simulink model "rfpsc_parallel"  (R2023b)
settings: Solver=VariableStepAuto  StartTime=0  StopTime=1.5  FixedStep=0.1*T_s  RelTol=1e-4  AbsTol=1e-4  EnableMultiTasking=on
StopFcn:
  | save('../converter-testing/sim.mat', 'u_c2', 'i_c2', 'u_c2_ref_lim', 'p_c2', 'q_c2', 'i_c2_ref', 'p_c2_ref', 'q_c2_ref', 'u_c1', 'i_c1', 'u_c1_ref_lim', 'p_c1', 'q_c1', 'i_c1_ref', 'p_c1_ref', 'q_c1_ref', 'u_pcc', 'i_g', 'u_hat_pcc', 'p_hat_g', 'q_hat_g', 'u_pcc_abc', 'i_g_abc', 'theta_g', 'theta_c2');
undefined symbols (not defined in the file): f_sw, K_p, kpp, L_f1, L_f2, L_g, R_a, R_f, R_f1, R_f2, R_L, T_s, U_dc, u_gN, w0_pll, w_b, w_g, w_N
libraries: simulink x2
settings Model: Creator=mhinkkan  LastModifiedBy=chowd
settings SolverCC: AutoScaleAbsTol=off  MaxConsecutiveMinStep=10  AlgebraicLoopSolver=TrustRegion
settings DataIOCC: SaveFormat=Array  SignalLoggingSaveFormat=ModelDataLogs  SaveOutput=off  SignalLogging=off  DSMLogging=off  ReturnWorkspaceOutputs=off
settings OptimizationCC: BlockReduction=off  BooleanDataType=off  DefaultParameterBehavior=Inlined  OptimizeBlockIOStorage=off  BufferReuse=off  ReuseModelBlockBuffer=off  ExpressionFolding=off  ExpressionDepthLimit=2147483647  LocalBlockOutputs=off  InitFltsAndDblsToZero=on  LifeSpan=inf
settings DebuggingCC: AlgebraicLoopMsg=none  SaveWithParameterizedLinksMsg=none  UnderspecifiedInitializationDetection=Classic  MergeDetectMultiDrivingBlocksExec=none  SignalResolutionControl=TryResolveAllWithWarning  MultiTaskDSMMsg=warning  MultiTaskCondExecSysMsg=none  FcnCallInpInsideContextMsg=warning  UnconnectedInputMsg=warning  UnconnectedOutputMsg=warning  UnconnectedLineMsg=warning  StateNameClashWarn=warning  SFUnexpectedBacktrackingDiag=warning  SFNoUnconditionalDefaultTransitionDiag=warning  SFExecutionAtInitializationDiag=none  ArithmeticOperatorsInVariantConditions=warning
settings HardwareCC: ProdBitPerPointer=32  ProdBitPerSizeT=32  ProdBitPerPtrDiffT=32  ProdLargestAtomicFloat=None  ProdIntDivRoundTo=Undefined  ProdEndianess=Unspecified  ProdWordSize=32  ProdHWDeviceType=32-bit Generic  TargetUnknown=on
settings ModelReferenceCC: PropagateSignalLabelsOutOfModel=off
settings SFSimCC: SimUseLocalCustomCode=off  CustomCodeUndefinedFunction=UseInterfaceOnly
settings RTWCC: RTWUseLocalCustomCode=off
settings CodeAppCC: StateflowObjectComments=on
settings GRTTargetCC: TargetFcnLib=ansi_tfl_tmw.mat  TargetLangStandard=C89/C90 (ANSI)  CombineOutputUpdateFcns=off  GRTInterface=on
settings ConfigComp: CovMetricSettings=dw  CovSaveCumulativeToWorkspaceVar=on  CovSaveSingleToWorkspaceVar=on  CovExternalEMLEnable=off

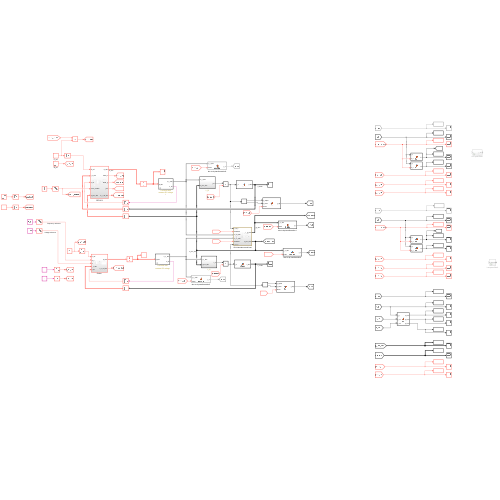
[thumbnail: Simulink's stored preview of the top-level diagram]
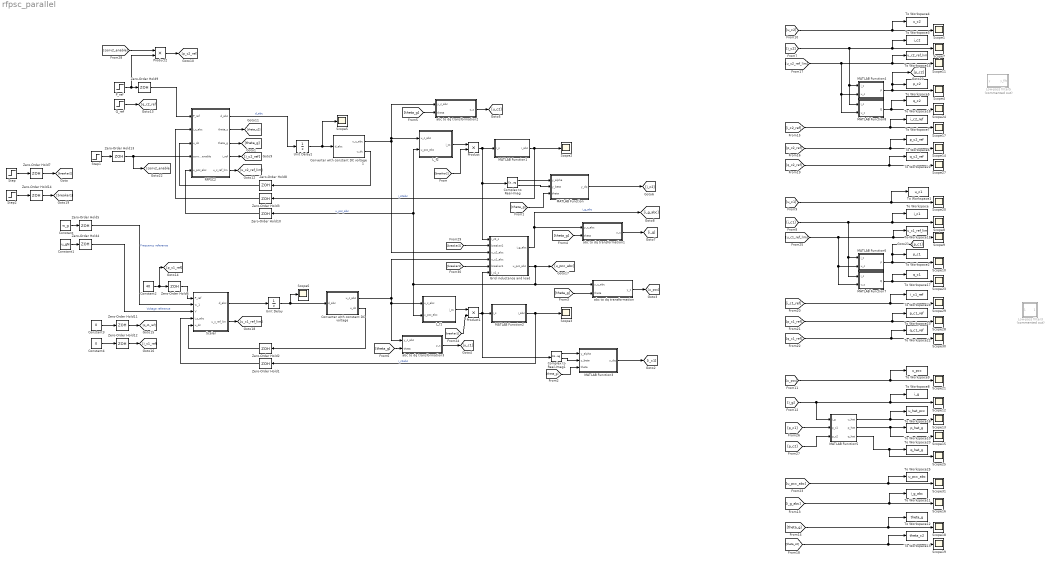
== system rfpsc_parallel ==
  Complex to Real-Imag : ComplexToRealImag
  Complex to Real-Imag1 : ComplexToRealImag
  Constant : Constant  Value=w_g
  Constant1 : Constant  Value=u_gN
  Constant2 : Constant  Value=40  SampleTime=T_s
  Constant3 : Constant  Value=0
  Constant4 : Constant  Value=0
  "Converter with constant DC voltage " : Subsystem  mask{f_sw=f_sw, u_dc=U_dc}
      mask prompts: f_sw "Switching frequency (Hz)"; u_dc "DC-bus voltage (V)"
      mask init:
      | T_s = 1/(2*f_sw);
  Converter with constant DC voltage 1 : Subsystem  mask{f_sw=f_sw, u_dc=U_dc}
      mask prompts: f_sw "Switching frequency (Hz)"; u_dc "DC-bus voltage (V)"
      mask init:
      | T_s = 1/(2*f_sw);
  Grid inductance and load : Subsystem
  L_f1 : Subsystem
  L_f2 : Subsystem
  Low-pass filter3 : Subsystem  Commented=on
  Low-pass filter5 : Subsystem  Commented=on
  MATLAB Function : MATLAB Function  TreatAsAtomicUnit=on
  MATLAB Function1 : MATLAB Function  TreatAsAtomicUnit=on
  MATLAB Function2 : MATLAB Function  TreatAsAtomicUnit=on
  MATLAB Function3 : MATLAB Function  TreatAsAtomicUnit=on
  MATLAB Function4 : MATLAB Function  TreatAsAtomicUnit=on
  MATLAB Function5 : MATLAB Function  TreatAsAtomicUnit=on
  MATLAB Function6 : MATLAB Function  TreatAsAtomicUnit=on
  MATLAB Function7 : MATLAB Function  TreatAsAtomicUnit=on
  MATLAB Function8 : MATLAB Function  TreatAsAtomicUnit=on
  P_ref : Step  Time=.9  Before=10  After=20  SampleTime=T_s
  Product : Product
  Product1 : Product
  Product2 : Product
  Q_ref : Step  Time=.35  After=0  SampleTime=T_s
  RFPSC2 : Subsystem
  "Scaler " : Subsystem
  Scope{1..21,23..25,27..31} (29 alike) : Scope
  Step : Step  Time=.3  SampleTime=T_s
  Step1 : Step  Time=.6  SampleTime=T_s
  Step2 : Step  Time=1.2  Before=1  After=0  SampleTime=T_s
  To Workspace : ToWorkspace  VariableName=i_c1  SaveFormat=Timeseries  SampleTime=-1
  To Workspace1 : ToWorkspace  VariableName=u_c1  SaveFormat=Timeseries  SampleTime=-1
  To Workspace10 : ToWorkspace  VariableName=p_hat_g  SaveFormat=Timeseries  SampleTime=-1
  To Workspace11 : ToWorkspace  VariableName=i_g_abc  SaveFormat=Timeseries  SampleTime=-1
  To Workspace12 : ToWorkspace  VariableName=theta_g  SaveFormat=Timeseries  SampleTime=-1
  To Workspace13 : ToWorkspace  VariableName=theta_c2  SaveFormat=Timeseries  SampleTime=-1
  To Workspace14 : ToWorkspace  VariableName=u_c2_ref_lim  SaveFormat=Timeseries  SampleTime=-1
  To Workspace15 : ToWorkspace  VariableName=u_c1_ref_lim  SaveFormat=Timeseries  SampleTime=-1
  To Workspace16 : ToWorkspace  VariableName=u_hat_pcc  SaveFormat=Timeseries  SampleTime=-1
  To Workspace17 : ToWorkspace  VariableName=q_c1  SaveFormat=Timeseries  SampleTime=-1
  To Workspace18 : ToWorkspace  VariableName=q_c2  SaveFormat=Timeseries  SampleTime=-1
  To Workspace2 : ToWorkspace  VariableName=p_c1  SaveFormat=Timeseries  SampleTime=-1
  To Workspace20 : ToWorkspace  VariableName=q_hat_g  SaveFormat=Timeseries  SampleTime=-1
  To Workspace21 : ToWorkspace  VariableName=q_c2_ref  SaveFormat=Timeseries  SampleTime=-1
  To Workspace22 : ToWorkspace  VariableName=q_c1_ref  SaveFormat=Timeseries  SampleTime=-1
  To Workspace23 : ToWorkspace  VariableName=p_c1_ref  SaveFormat=Timeseries  SampleTime=-1
  To Workspace24 : ToWorkspace  VariableName=i_c1_ref  SaveFormat=Timeseries  SampleTime=-1
  To Workspace25 : ToWorkspace  VariableName=u_pcc_abc  SaveFormat=Timeseries  SampleTime=-1
  To Workspace3 : ToWorkspace  VariableName=i_c2  SaveFormat=Timeseries  SampleTime=-1
  To Workspace4 : ToWorkspace  VariableName=u_c2  SaveFormat=Timeseries  SampleTime=-1
  To Workspace5 : ToWorkspace  VariableName=p_c2  SaveFormat=Timeseries  SampleTime=-1
  To Workspace6 : ToWorkspace  VariableName=p_c2_ref  SaveFormat=Timeseries  SampleTime=-1
  To Workspace7 : ToWorkspace  VariableName=i_c2_ref  SaveFormat=Timeseries  SampleTime=-1
  To Workspace8 : ToWorkspace  VariableName=i_g  SaveFormat=Timeseries  SampleTime=-1
  To Workspace9 : ToWorkspace  VariableName=u_pcc  SaveFormat=Timeseries  SampleTime=-1
  Unit Delay : UnitDelay  SampleTime=T_s  HasFrameUpgradeWarning=on
  Unit Delay1 : UnitDelay  SampleTime=T_s  HasFrameUpgradeWarning=on
  Zero-Order Hold{1..14} (14 alike) : ZeroOrderHold  SampleTime=T_s
  abc to dq transformation : MATLAB Function  TreatAsAtomicUnit=on
  abc to dq transformation1 : MATLAB Function  TreatAsAtomicUnit=on
  abc to dq transformation2 : MATLAB Function  TreatAsAtomicUnit=on
  abc to dq transformation3 : MATLAB Function  TreatAsAtomicUnit=on
  wires:
  Grid inductance and load/1(i_g_abc) -> [i_g_abc], abc to dq transformation1/1(y_c_abc)  "i_g_abc"
  Product1/1 -> Grid inductance and load/6(i_c1_s), Complex to Real-Imag1/1, MATLAB Function2/1(i_s)
  MATLAB Function2/1(i_abc) -> Scope3/1, Zero-Order Hold1/1  "i_c1abc"
  Grid inductance and load/2(u_pcc_abc) -> Zero-Order Hold10/1, L_f2/2(u_pcc_abc), L_f1/2(u_pcc_abc), abc to dq transformation/1(y_c_abc), [u_pcc_abc]  "u_pcc_abc"
  "Converter with constant DC voltage "/2(u_dc) -> Zero-Order Hold2/1
  "Scaler "/1(d_abc) -> Unit Delay/1
  Zero-Order Hold4/1 -> "Scaler "/3(V)  "Voltage reference"
  Constant1/1 -> Zero-Order Hold4/1
  Unit Delay/1 -> "Converter with constant DC voltage "/1(d_abc), Scope6/1
  Constant/1 -> Zero-Order Hold5/1
  Zero-Order Hold5/1 -> "Scaler "/2(w_1)  "Frequency reference"
  "Converter with constant DC voltage "/1(u_c_abc) -> abc to dq transformation3/1(y_c_abc), L_f1/1(u_c_abc), Grid inductance and load/4(u_c1_abc)
  Converter with constant DC voltage 1/1(u_c_abc) -> L_f2/1(u_c_abc), abc to dq transformation2/1(y_c_abc), Grid inductance and load/3(u_c2_abc)
  Unit Delay1/1 -> Scope5/1, Converter with constant DC voltage 1/1(d_abc)
  P_ref/1 -> Zero-Order Hold9/1, Product2/2
  Zero-Order Hold9/1 -> RFPSC2/1(P_ref)
  Converter with constant DC voltage 1/2(u_dc) -> Zero-Order Hold8/1
  MATLAB Function1/1(i_abc) -> Zero-Order Hold3/1, Scope2/1  "i_c2abc"
  Zero-Order Hold8/1 -> RFPSC2/3(u_dc)
  Zero-Order Hold3/1 -> RFPSC2/2(i_c_abc)
  Zero-Order Hold2/1 -> "Scaler "/5(u_dc)
  Zero-Order Hold1/1 -> "Scaler "/4(i_c_abc)
  Constant2/1 -> [p_c1_ref], Zero-Order Hold6/1
  Zero-Order Hold6/1 -> "Scaler "/1(P_ref)
  Step/1 -> Zero-Order Hold7/1
  Zero-Order Hold7/1 -> [breaker2]
  RFPSC2/1(d_abc) -> Unit Delay1/1  "d_abc"
  Product/1 -> Complex to Real-Imag/1, Grid inductance and load/1(i_c2_s), MATLAB Function1/1(i_s)
  L_f2/1(i_cs) -> Product/1
  [breaker2] -> Product/2
  Complex to Real-Imag/1 -> MATLAB Function/1(y_alpha)
  Complex to Real-Imag/2 -> MATLAB Function/2(y_beta)
  [theta_g] -> MATLAB Function/3(theta)
  Complex to Real-Imag1/1 -> MATLAB Function3/1(y_alpha)
  Complex to Real-Imag1/2 -> MATLAB Function3/2(y_beta)
  [theta_g] -> MATLAB Function3/3(theta)
  MATLAB Function3/1(y_dq) -> [i_c1]
  [theta_g] -> abc to dq transformation/2(theta)
  [theta_g] -> abc to dq transformation1/2(theta)
  [theta_g] -> abc to dq transformation2/2(theta)
  [theta_g] -> abc to dq transformation3/2(theta)
  Zero-Order Hold10/1 -> RFPSC2/5(u_pcc_abc)
  RFPSC2/3(theta_g) -> [theta_g]
  abc to dq transformation/1(y_c) -> [u_pcc]
  abc to dq transformation3/1(y_c) -> [u_c1]
  abc to dq transformation2/1(y_c) -> [u_c2]
  MATLAB Function/1(y_dq) -> [i_c2]
  abc to dq transformation1/1(y_c) -> [i_g]
  [i_c1] -> To Workspace/1, Scope8/1, MATLAB Function7/1(i_c), MATLAB Function6/1(i_c)
  RFPSC2/4(i_ref) -> [i_c2_ref]
  RFPSC2/2(theta_c) -> [theta_c2]
  RFPSC2/5(u_c_ref_lim) -> [u_c2_ref_lim]
  MATLAB Function6/1(P) -> To Workspace2/1, [p_c1], Scope10/1
  MATLAB Function4/1(P) -> [p_c2], To Workspace5/1, Scope4/1
  [i_c2] -> To Workspace3/1, Scope7/1, MATLAB Function8/1(i_c), MATLAB Function4/1(i_c)
  [p_c2_ref] -> To Workspace6/1, Scope14/1
  MATLAB Function5/2(p_hat) -> Scope15/1, To Workspace10/1
  [i_g_abc] -> To Workspace11/1, Scope16/1
  [i_c2_ref] -> To Workspace7/1, Scope17/1
  [theta_g] -> To Workspace12/1, Scope18/1
  [theta_c2] -> To Workspace13/1, Scope19/1
  MATLAB Function7/1(Q) -> To Workspace17/1, Scope23/1
  MATLAB Function8/1(Q) -> To Workspace18/1, Scope24/1
  MATLAB Function5/3(q_hat) -> Scope25/1, To Workspace20/1
  Q_ref/1 -> [q_c2_ref]
  [q_c2_ref] -> To Workspace21/1, Scope27/1
  [q_c1_ref] -> Scope30/1, To Workspace22/1
  [i_c1_ref] -> Scope29/1, To Workspace24/1
  [p_c1_ref] -> Scope28/1, To Workspace23/1
  Constant3/1 -> Zero-Order Hold11/1
  Constant4/1 -> Zero-Order Hold12/1
  [u_c1_ref_lim] -> To Workspace15/1, Scope9/1, MATLAB Function6/2(u_c), MATLAB Function7/2(u_c)
  [u_c2_ref_lim] -> To Workspace14/1, Scope11/1, MATLAB Function8/2(u_c), MATLAB Function4/2(u_c)
  [u_pcc_abc] -> To Workspace25/1, Scope31/1
  Zero-Order Hold11/1 -> [q_c1_ref]
  Zero-Order Hold12/1 -> [i_c1_ref]
  "Scaler "/2(u_c_ref_lim) -> [u_c1_ref_lim]
  Step1/1 -> Zero-Order Hold13/1
  Zero-Order Hold13/1 -> [conv2_enable], RFPSC2/4(conv_enable)
  Zero-Order Hold14/1 -> [breaker1]
  Step2/1 -> Zero-Order Hold14/1
  L_f1/1(i_cs) -> Product1/1
  [breaker1] -> Product1/2
  [u_c2] -> To Workspace4/1, Scope1/1
  [u_c1] -> To Workspace1/1, Scope20/1
  [u_pcc] -> Scope21/1, To Workspace9/1
  [i_g] -> MATLAB Function5/1(i_g), To Workspace8/1, Scope12/1
  MATLAB Function5/1(u_hat) -> To Workspace16/1, Scope13/1
  [p_c1] -> MATLAB Function5/2(p_c1)
  [p_c2] -> MATLAB Function5/3(p_c2)
  [conv2_enable] -> Product2/1
  Product2/1 -> [p_c2_ref]
  [breaker2] -> Grid inductance and load/2(breaker2)
  [breaker1] -> Grid inductance and load/5(breaker1)

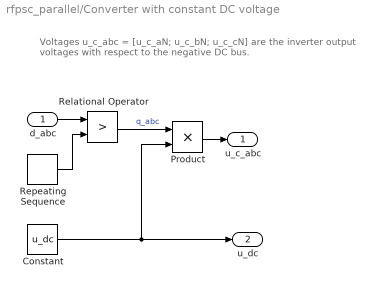
== system rfpsc_parallel/Converter with constant DC voltage  ==
  note: Voltages u_c_abc = [u_c_aN; u_c_bN; u_c_cN] are the inverter
      | output voltages with respect to the negative DC bus.
  d_abc : Inport
  Constant : Constant  Value=u_dc
  Product : Product
  Relational Operator : RelationalOperator  Operator=>  OutDataTypeStr='double'  InputSameDT=off
  Repeating Sequence : simulink/Sources/Repeating Sequence  rep_seq_t=[0 1 2]*T_s  rep_seq_y=[1 0 1]
  u_c_abc : Outport
  u_dc : Outport  Port=2
  wires:
  Repeating Sequence/1 -> Relational Operator/2
  d_abc/1 -> Relational Operator/1
  Product/1 -> u_c_abc/1
  Relational Operator/1 -> Product/1  "q_abc"
  Constant/1 -> Product/2, u_dc/1

== system rfpsc_parallel/Converter with constant DC voltage 1 ==
  note: Voltages u_c_abc = [u_c_aN; u_c_bN; u_c_cN] are the inverter
      | output voltages with respect to the negative DC bus.
  d_abc : Inport
  Constant : Constant  Value=u_dc
  Product : Product
  Relational Operator : RelationalOperator  Operator=>  OutDataTypeStr='double'  InputSameDT=off
  Repeating Sequence : simulink/Sources/Repeating Sequence  rep_seq_t=[0 1 2]*T_s  rep_seq_y=[1 0 1]
  u_c_abc : Outport
  u_dc : Outport  Port=2
  wires:
  Constant/1 -> u_dc/1, Product/2
  Relational Operator/1 -> Product/1  "q_abc"
  Product/1 -> u_c_abc/1
  d_abc/1 -> Relational Operator/1
  Repeating Sequence/1 -> Relational Operator/2

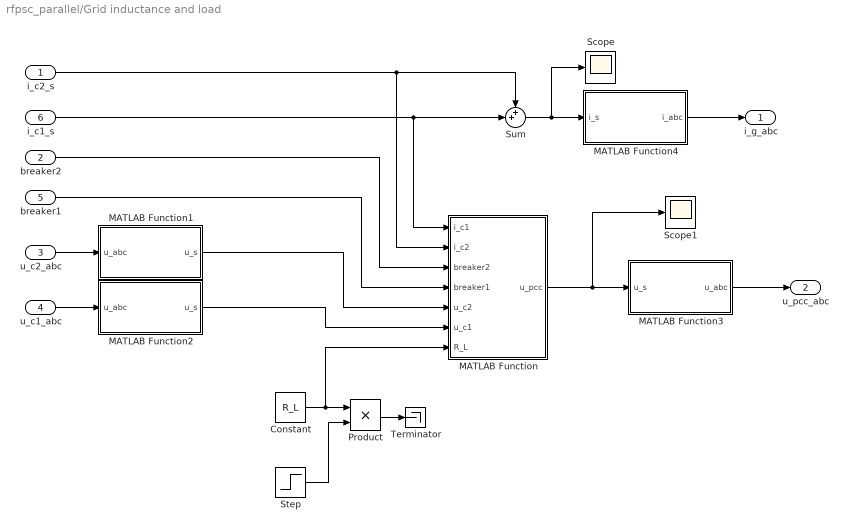
== system rfpsc_parallel/Grid inductance and load ==
  i_c2_s : Inport
  breaker2 : Inport  Port=2
  u_c2_abc : Inport  Port=3
  u_c1_abc : Inport  Port=4
  breaker1 : Inport  Port=5
  i_c1_s : Inport  Port=6
  Constant : Constant  Value=R_L  SampleTime=-1
  MATLAB Function : MATLAB Function  TreatAsAtomicUnit=on
  MATLAB Function1 : MATLAB Function  TreatAsAtomicUnit=on
  MATLAB Function2 : MATLAB Function  TreatAsAtomicUnit=on
  MATLAB Function3 : MATLAB Function  TreatAsAtomicUnit=on
  MATLAB Function4 : MATLAB Function  TreatAsAtomicUnit=on
  Product : Product
  Scope : Scope
  Scope1 : Scope
  Step : Step  Time=.06  Before=1  After=0.5  SampleTime=T_s
  Sum : Sum  Inputs=++|
  Terminator : Terminator
  i_g_abc : Outport
  u_pcc_abc : Outport  Port=2
  wires:
  Sum/1 -> MATLAB Function4/1(i_s), Scope/1
  i_c2_s/1 -> Sum/1, MATLAB Function/2(i_c2)
  i_c1_s/1 -> MATLAB Function/1(i_c1), Sum/2
  u_c2_abc/1 -> MATLAB Function1/1(u_abc)
  u_c1_abc/1 -> MATLAB Function2/1(u_abc)
  MATLAB Function1/1(u_s) -> MATLAB Function/5(u_c2)
  MATLAB Function2/1(u_s) -> MATLAB Function/6(u_c1)
  MATLAB Function/1(u_pcc) -> Scope1/1, MATLAB Function3/1(u_s)
  MATLAB Function3/1(u_abc) -> u_pcc_abc/1
  MATLAB Function4/1(i_abc) -> i_g_abc/1
  Step/1 -> Product/2
  Constant/1 -> MATLAB Function/7(R_L), Product/1
  Product/1 -> Terminator/1
  breaker2/1 -> MATLAB Function/3(breaker2)
  breaker1/1 -> MATLAB Function/4(breaker1)

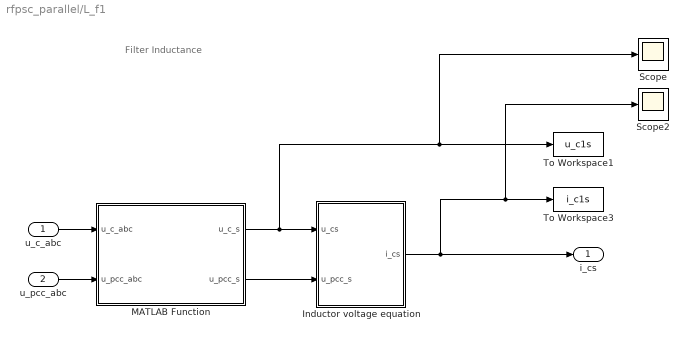
== system rfpsc_parallel/L_f1 ==
  note: Filter Inductance
  u_c_abc : Inport
  u_pcc_abc : Inport  Port=2
  Inductor voltage equation : Subsystem
  MATLAB Function : MATLAB Function  TreatAsAtomicUnit=on
  Scope : Scope
  Scope2 : Scope
  To Workspace1 : ToWorkspace  VariableName=u_c1s  SaveFormat=Timeseries
  To Workspace3 : ToWorkspace  VariableName=i_c1s  SaveFormat=Timeseries
  i_cs : Outport
  wires:
  Inductor voltage equation/1(i_cs) -> i_cs/1, Scope2/1, To Workspace3/1
  MATLAB Function/1(u_c_s) -> Inductor voltage equation/1(u_cs), Scope/1, To Workspace1/1
  u_c_abc/1 -> MATLAB Function/1(u_c_abc)
  MATLAB Function/2(u_pcc_s) -> Inductor voltage equation/2(u_pcc_s)
  u_pcc_abc/1 -> MATLAB Function/2(u_pcc_abc)

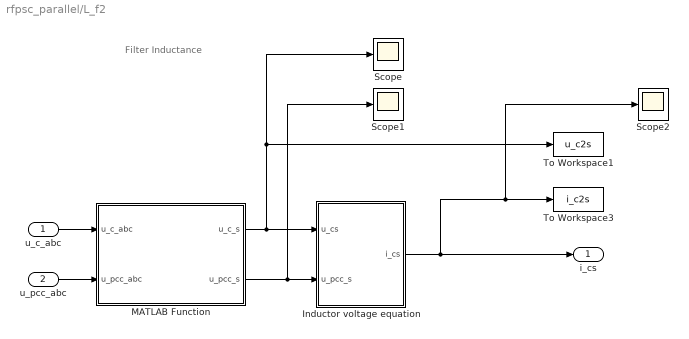
== system rfpsc_parallel/L_f2 ==
  note: Filter Inductance
  u_c_abc : Inport
  u_pcc_abc : Inport  Port=2
  Inductor voltage equation : Subsystem
  MATLAB Function : MATLAB Function  TreatAsAtomicUnit=on
  Scope : Scope
  Scope1 : Scope
  Scope2 : Scope
  To Workspace1 : ToWorkspace  VariableName=u_c2s  SaveFormat=Timeseries
  To Workspace3 : ToWorkspace  VariableName=i_c2s  SaveFormat=Timeseries
  i_cs : Outport
  wires:
  Inductor voltage equation/1(i_cs) -> i_cs/1, Scope2/1, To Workspace3/1
  MATLAB Function/1(u_c_s) -> Inductor voltage equation/1(u_cs), To Workspace1/1, Scope/1
  u_c_abc/1 -> MATLAB Function/1(u_c_abc)
  MATLAB Function/2(u_pcc_s) -> Scope1/1, Inductor voltage equation/2(u_pcc_s)
  u_pcc_abc/1 -> MATLAB Function/2(u_pcc_abc)

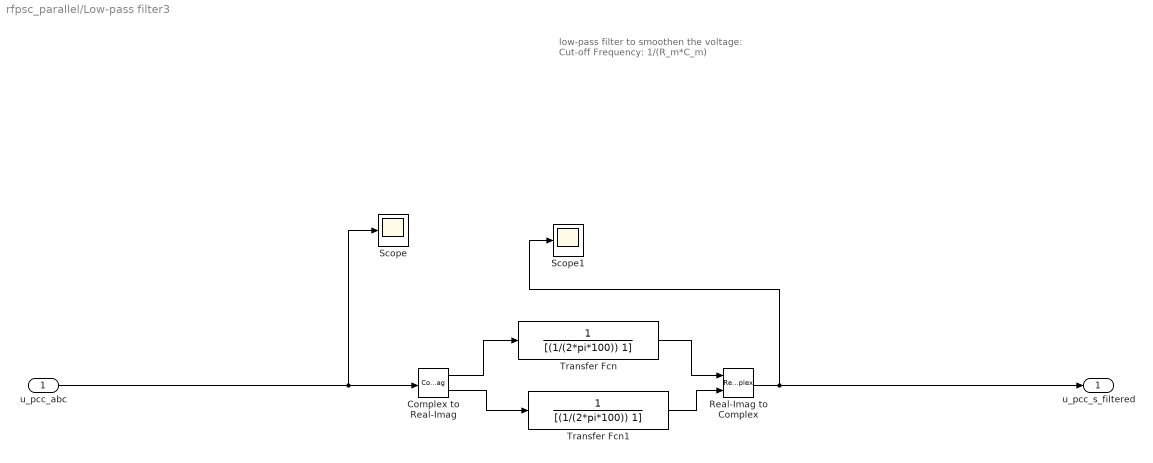
== system rfpsc_parallel/Low-pass filter3 ==
  note: low-pass filter to smoothen the voltage:
      | Cut-off Frequency: 1/(R_m*C_m)
  u_pcc_abc : Inport
  Complex to Real-Imag : ComplexToRealImag
  Real-Imag to Complex : RealImagToComplex
  Scope : Scope
  Scope1 : Scope
  Transfer Fcn : TransferFcn  Denominator=[(1/(2*pi*100)) 1]
  Transfer Fcn1 : TransferFcn  Denominator=[(1/(2*pi*100)) 1]
  u_pcc_s_filtered : Outport
  wires:
  Transfer Fcn1/1 -> Real-Imag to Complex/2
  Real-Imag to Complex/1 -> u_pcc_s_filtered/1, Scope1/1
  Complex to Real-Imag/1 -> Transfer Fcn/1
  u_pcc_abc/1 -> Complex to Real-Imag/1, Scope/1
  Transfer Fcn/1 -> Real-Imag to Complex/1
  Complex to Real-Imag/2 -> Transfer Fcn1/1

== system rfpsc_parallel/Low-pass filter5 ==
  note: low-pass filter to smoothen the voltage:
      | Cut-off Frequency: 1/(R_m*C_m)
  y : Inport
  Complex to Real-Imag : ComplexToRealImag
  Real-Imag to Complex : RealImagToComplex
  Transfer Fcn : TransferFcn  Denominator=[(1/(2*pi*1100)) 1]
  Transfer Fcn1 : TransferFcn  Denominator=[(1/(2*pi*1100)) 1]
  y_filt : Outport
  wires:
  Real-Imag to Complex/1 -> y_filt/1
  y/1 -> Complex to Real-Imag/1
  Transfer Fcn/1 -> Real-Imag to Complex/2
  Transfer Fcn1/1 -> Real-Imag to Complex/1
  Complex to Real-Imag/2 -> Transfer Fcn/1
  Complex to Real-Imag/1 -> Transfer Fcn1/1

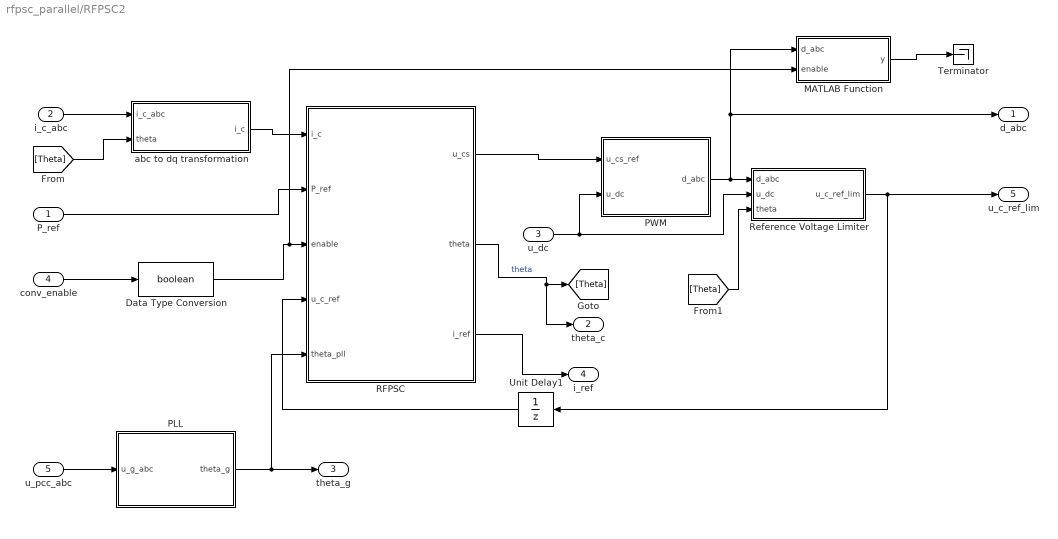
== system rfpsc_parallel/RFPSC2 ==
  P_ref : Inport
  i_c_abc : Inport  Port=2
  u_dc : Inport  Port=3
  conv_enable : Inport  Port=4
  u_pcc_abc : Inport  Port=5
  Data Type Conversion : DataTypeConversion  OutDataTypeStr=boolean  SaturateOnIntegerOverflow=off  RndMeth=Floor
  MATLAB Function : MATLAB Function  TreatAsAtomicUnit=on
  PLL : Subsystem
  PWM : Subsystem
  RFPSC : Subsystem
  Reference Voltage Limiter : Subsystem
  Terminator : Terminator
  Unit Delay1 : UnitDelay  SampleTime=T_s  HasFrameUpgradeWarning=on
  abc to dq transformation : MATLAB Function  TreatAsAtomicUnit=on  SystemSampleTime=T_s
  d_abc : Outport
  theta_c : Outport  Port=2
  theta_g : Outport  Port=3
  i_ref : Outport  Port=4
  u_c_ref_lim : Outport  Port=5
  wires:
  conv_enable/1 -> Data Type Conversion/1
  [Theta] -> Reference Voltage Limiter/3(theta)
  PWM/1(d_abc) -> d_abc/1, MATLAB Function/1(d_abc), Reference Voltage Limiter/1(d_abc)
  RFPSC/1(u_cs) -> PWM/1(u_cs_ref)
  Unit Delay1/1 -> RFPSC/4(u_c_ref)
  P_ref/1 -> RFPSC/2(P_ref)
  abc to dq transformation/1(i_c) -> RFPSC/1(i_c)
  Reference Voltage Limiter/1(u_c_ref_lim) -> Unit Delay1/1, u_c_ref_lim/1
  u_dc/1 -> Reference Voltage Limiter/2(u_dc), PWM/2(u_dc)
  [Theta] -> abc to dq transformation/2(theta)
  RFPSC/2(theta) -> theta_c/1, [Theta]  "theta"
  i_c_abc/1 -> abc to dq transformation/1(i_c_abc)
  PLL/1(theta_g) -> RFPSC/5(theta_pll), theta_g/1
  u_pcc_abc/1 -> PLL/1(u_g_abc)
  Data Type Conversion/1 -> MATLAB Function/2(enable), RFPSC/3(enable)
  MATLAB Function/1(y) -> Terminator/1
  RFPSC/3(i_ref) -> i_ref/1

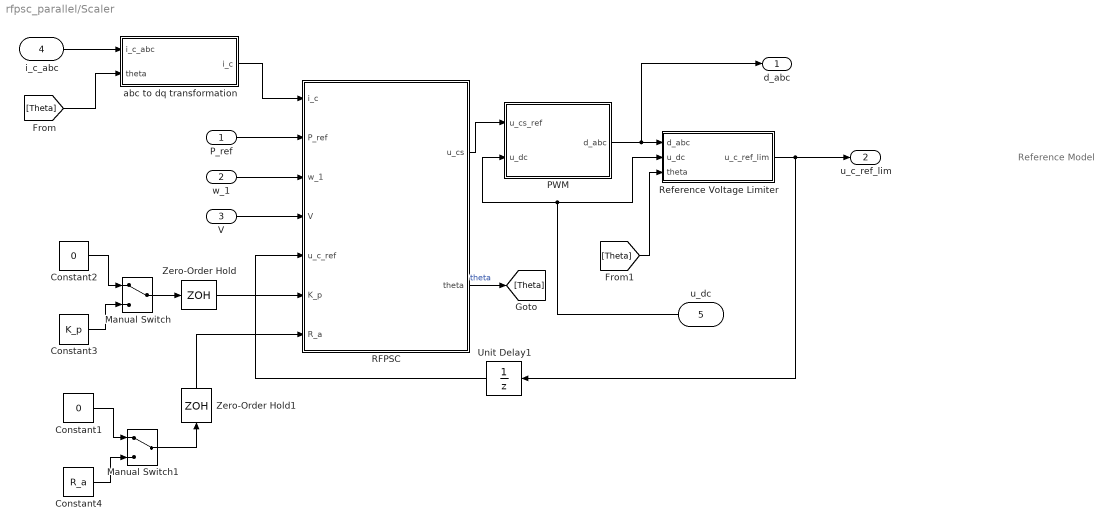
== system rfpsc_parallel/Scaler  ==
  note: Reference Model
  P_ref : Inport
  w_1 : Inport  Port=2
  V : Inport  Port=3
  i_c_abc : Inport  Port=4
  u_dc : Inport  Port=5
  Constant1 : Constant  Value=0  SampleTime=T_s
  Constant2 : Constant  Value=0  SampleTime=T_s
  Constant3 : Constant  Value=K_p  SampleTime=T_s
  Constant4 : Constant  Value=R_a  SampleTime=T_s
  Manual Switch : ManualSwitch
  Manual Switch1 : ManualSwitch
  PWM : Subsystem
  RFPSC : Subsystem
  Reference Voltage Limiter : Subsystem
  Unit Delay1 : UnitDelay  SampleTime=-1  HasFrameUpgradeWarning=on
  Zero-Order Hold : ZeroOrderHold  SampleTime=T_s
  Zero-Order Hold1 : ZeroOrderHold  SampleTime=T_s
  abc to dq transformation : MATLAB Function  TreatAsAtomicUnit=on
  d_abc : Outport
  u_c_ref_lim : Outport  Port=2
  wires:
  w_1/1 -> RFPSC/3(w_1)
  abc to dq transformation/1(i_c) -> RFPSC/1(i_c)
  Unit Delay1/1 -> RFPSC/5(u_c_ref)
  [Theta] -> abc to dq transformation/2(theta)
  [Theta] -> Reference Voltage Limiter/3(theta)
  Reference Voltage Limiter/1(u_c_ref_lim) -> Unit Delay1/1, u_c_ref_lim/1
  P_ref/1 -> RFPSC/2(P_ref)
  i_c_abc/1 -> abc to dq transformation/1(i_c_abc)
  PWM/1(d_abc) -> d_abc/1, Reference Voltage Limiter/1(d_abc)
  V/1 -> RFPSC/4(V)
  u_dc/1 -> PWM/2(u_dc), Reference Voltage Limiter/2(u_dc)
  RFPSC/1(u_cs) -> PWM/1(u_cs_ref)
  RFPSC/2(theta) -> [Theta]  "theta"
  Constant4/1 -> Manual Switch1/2
  Constant2/1 -> Manual Switch/1
  Manual Switch1/1 -> Zero-Order Hold1/1
  Constant1/1 -> Manual Switch1/1
  Constant3/1 -> Manual Switch/2
  Manual Switch/1 -> Zero-Order Hold/1
  Zero-Order Hold/1 -> RFPSC/6(K_p)
  Zero-Order Hold1/1 -> RFPSC/7(R_a)

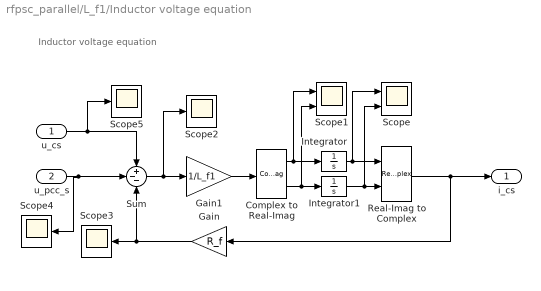
== system rfpsc_parallel/L_f1/Inductor voltage equation ==
  note: Inductor voltage equation
  u_cs : Inport
  u_pcc_s : Inport  Port=2
  Complex to Real-Imag : ComplexToRealImag
  Gain : Gain  Gain=R_f
  Gain1 : Gain  Gain=1/L_f1
  Integrator : Integrator
  Integrator1 : Integrator
  Real-Imag to Complex : RealImagToComplex
  Scope : Scope  NumInputPorts=2
  Scope1 : Scope  NumInputPorts=2
  Scope{2..5} (4 alike) : Scope
  Sum : Sum  Inputs=+--
  i_cs : Outport
  wires:
  Gain/1 -> Scope3/1, Sum/3
  Real-Imag to Complex/1 -> i_cs/1, Gain/1
  Integrator1/1 -> Real-Imag to Complex/2, Scope/2
  Integrator/1 -> Real-Imag to Complex/1, Scope/1
  Complex to Real-Imag/2 -> Integrator1/1, Scope1/2
  Complex to Real-Imag/1 -> Integrator/1, Scope1/1
  Gain1/1 -> Complex to Real-Imag/1
  Sum/1 -> Scope2/1, Gain1/1
  u_pcc_s/1 -> Scope4/1, Sum/2
  u_cs/1 -> Scope5/1, Sum/1

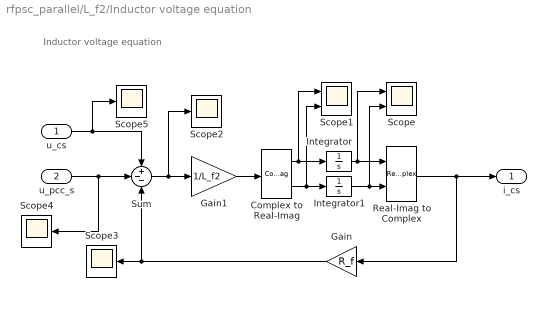
== system rfpsc_parallel/L_f2/Inductor voltage equation ==
  note: Inductor voltage equation
  u_cs : Inport
  u_pcc_s : Inport  Port=2
  Complex to Real-Imag : ComplexToRealImag
  Gain : Gain  Gain=R_f
  Gain1 : Gain  Gain=1/L_f2
  Integrator : Integrator
  Integrator1 : Integrator
  Real-Imag to Complex : RealImagToComplex
  Scope : Scope  NumInputPorts=2
  Scope1 : Scope  NumInputPorts=2
  Scope{2..5} (4 alike) : Scope
  Sum : Sum  Inputs=+--
  i_cs : Outport
  wires:
  Gain/1 -> Sum/3, Scope3/1
  Real-Imag to Complex/1 -> Gain/1, i_cs/1
  Integrator1/1 -> Real-Imag to Complex/2, Scope/2
  Integrator/1 -> Real-Imag to Complex/1, Scope/1
  Complex to Real-Imag/2 -> Integrator1/1, Scope1/2
  Complex to Real-Imag/1 -> Integrator/1, Scope1/1
  Gain1/1 -> Complex to Real-Imag/1
  Sum/1 -> Scope2/1, Gain1/1
  u_pcc_s/1 -> Scope4/1, Sum/2
  u_cs/1 -> Scope5/1, Sum/1

== system rfpsc_parallel/RFPSC2/PLL ==
  u_g_abc : Inport
  PLL : MATLAB Function  TreatAsAtomicUnit=on  SystemSampleTime=T_s
  Unit Delay : UnitDelay  InitialCondition=w_N  SampleTime=T_s  HasFrameUpgradeWarning=on
  Unit Delay1 : UnitDelay  SampleTime=T_s  HasFrameUpgradeWarning=on
  theta_g : Outport
  wires:
  u_g_abc/1 -> PLL/1(u_g_abc)
  PLL/2(w_gi_new) -> Unit Delay/1
  PLL/1(theta_g_new) -> Unit Delay1/1
  Unit Delay1/1 -> PLL/2(theta_g), theta_g/1
  Unit Delay/1 -> PLL/3(w_gi)

== system rfpsc_parallel/RFPSC2/PWM ==
  u_cs_ref : Inport
  u_dc : Inport  Port=2
  MATLAB Function : MATLAB Function  TreatAsAtomicUnit=on  SystemSampleTime=T_s
  d_abc : Outport  OutDataTypeStr=double
  wires:
  MATLAB Function/1(d_abc) -> d_abc/1
  u_dc/1 -> MATLAB Function/2(u_dc)
  u_cs_ref/1 -> MATLAB Function/1(u_cs_ref)

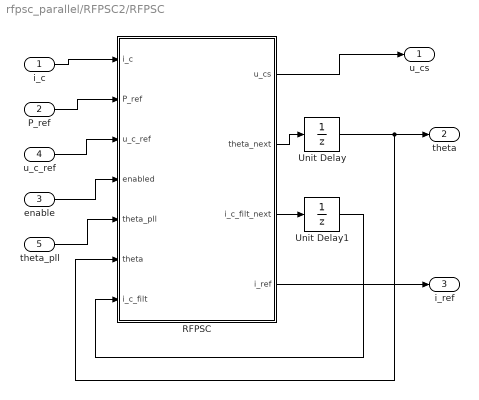
== system rfpsc_parallel/RFPSC2/RFPSC ==
  i_c : Inport
  P_ref : Inport  Port=2
  enable : Inport  Port=3
  u_c_ref : Inport  Port=4
  theta_pll : Inport  Port=5
  RFPSC : MATLAB Function  TreatAsAtomicUnit=on  SystemSampleTime=T_s
  Unit Delay : UnitDelay  SampleTime=T_s  HasFrameUpgradeWarning=on
  Unit Delay1 : UnitDelay  SampleTime=T_s  HasFrameUpgradeWarning=on
  u_cs : Outport  OutDataTypeStr=double
      settings: SignalType=complex
  theta : Outport  Port=2  OutDataTypeStr=double
  i_ref : Outport  Port=3
  wires:
  enable/1 -> RFPSC/4(enabled)
  Unit Delay1/1 -> RFPSC/7(i_c_filt)
  RFPSC/3(i_c_filt_next) -> Unit Delay1/1
  Unit Delay/1 -> theta/1, RFPSC/6(theta)
  u_c_ref/1 -> RFPSC/3(u_c_ref)
  i_c/1 -> RFPSC/1(i_c)
  P_ref/1 -> RFPSC/2(P_ref)
  RFPSC/2(theta_next) -> Unit Delay/1
  RFPSC/1(u_cs) -> u_cs/1
  theta_pll/1 -> RFPSC/5(theta_pll)
  RFPSC/4(i_ref) -> i_ref/1

== system rfpsc_parallel/RFPSC2/Reference Voltage Limiter ==
  d_abc : Inport
  u_dc : Inport  Port=2
  theta : Inport  Port=3
  MATLAB Function : MATLAB Function  TreatAsAtomicUnit=on  SystemSampleTime=T_s
  u_c_ref_lim : Outport
  wires:
  u_dc/1 -> MATLAB Function/2(u_dc)
  MATLAB Function/1(u_c_ref_lim) -> u_c_ref_lim/1
  theta/1 -> MATLAB Function/3(theta)
  d_abc/1 -> MATLAB Function/1(d_abc)

== system rfpsc_parallel/Scaler /PWM ==
  u_cs_ref : Inport
  u_dc : Inport  Port=2
  MATLAB Function : MATLAB Function  TreatAsAtomicUnit=on
  d_abc : Outport
  wires:
  u_cs_ref/1 -> MATLAB Function/1(u_cs_ref)
  u_dc/1 -> MATLAB Function/2(u_dc)
  MATLAB Function/1(d_abc) -> d_abc/1

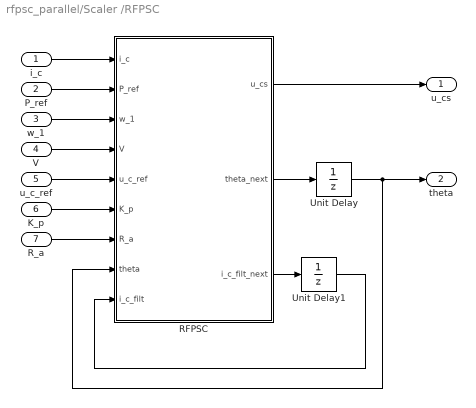
== system rfpsc_parallel/Scaler /RFPSC ==
  i_c : Inport
  P_ref : Inport  Port=2
  w_1 : Inport  Port=3
  V : Inport  Port=4
  u_c_ref : Inport  Port=5
  K_p : Inport  Port=6
  R_a : Inport  Port=7
  RFPSC : MATLAB Function  TreatAsAtomicUnit=on  SystemSampleTime=T_s
  Unit Delay : UnitDelay  SampleTime=T_s  HasFrameUpgradeWarning=on
  Unit Delay1 : UnitDelay  SampleTime=T_s  HasFrameUpgradeWarning=on
  u_cs : Outport  OutDataTypeStr=double
      settings: SignalType=complex
  theta : Outport  Port=2  OutDataTypeStr=double
  wires:
  Unit Delay1/1 -> RFPSC/9(i_c_filt)
  RFPSC/3(i_c_filt_next) -> Unit Delay1/1
  Unit Delay/1 -> theta/1, RFPSC/8(theta)
  u_c_ref/1 -> RFPSC/5(u_c_ref)
  w_1/1 -> RFPSC/3(w_1)
  i_c/1 -> RFPSC/1(i_c)
  P_ref/1 -> RFPSC/2(P_ref)
  V/1 -> RFPSC/4(V)
  RFPSC/2(theta_next) -> Unit Delay/1
  RFPSC/1(u_cs) -> u_cs/1
  K_p/1 -> RFPSC/6(K_p)
  R_a/1 -> RFPSC/7(R_a)

== system rfpsc_parallel/Scaler /Reference Voltage Limiter ==
  d_abc : Inport
  u_dc : Inport  Port=2
  theta : Inport  Port=3
  MATLAB Function : MATLAB Function  TreatAsAtomicUnit=on
  u_c_ref_lim : Outport
  wires:
  d_abc/1 -> MATLAB Function/1(d_abc)
  theta/1 -> MATLAB Function/3(theta)
  MATLAB Function/1(u_c_ref_lim) -> u_c_ref_lim/1
  u_dc/1 -> MATLAB Function/2(u_dc)

== matlab function rfpsc_parallel/RFPSC2/MATLAB Function ==
  data: d_abc input; y output; enable input
function y = fcn(d_abc, enable)

if(enable==1)
    y = d_abc;
else
    y = [0; 0; 0];
end

== matlab function rfpsc_parallel/MATLAB Function6 ==
  data: i_c input; u_c input; P output
function P = fcn(i_c, u_c)

P = 3/2*real((u_c)*conj(i_c));

== matlab function rfpsc_parallel/MATLAB Function ==
  data: y_alpha input double; y_dq output double; y_beta input double; theta input
function y_dq = fcn(y_alpha, y_beta, theta)

% Coordinate Transformation (Alpha-beta to dq)
y_s = y_alpha + 1j*y_beta;
y_dq = y_s * exp(-1j*theta);

== matlab function rfpsc_parallel/MATLAB Function1 ==
  data: i_s input size=1; i_abc output size=3
function i_abc = s2abc(i_s)

% Inverse space-vector transformation
i_abc = real([1; exp(-1j*2*pi/3); exp(-1j*4*pi/3)]*i_s);

== matlab function rfpsc_parallel/MATLAB Function2 ==
  data: i_s input size=1; i_abc output size=3
function i_abc = s2abc(i_s)

% Inverse space-vector transformation
i_abc = real([1; exp(-1j*2*pi/3); exp(-1j*4*pi/3)]*i_s);

== matlab function rfpsc_parallel/RFPSC2/RFPSC/RFPSC ==
  data: i_c input; P_ref input; u_cs output double; theta_next output; u_c_ref input; enabled input boolean; theta_pll input; theta input; i_c_filt input; K_p parameter; T_s parameter; R_a parameter; i_c_filt_next output double; w_b parameter; kpp parameter; w_N parameter; u_gN parameter; i_ref output
function [u_cs, theta_next, i_c_filt_next, i_ref] = ... 
    RFPSC(i_c, P_ref, u_c_ref, enabled, theta_pll, theta, i_c_filt, ... 
    K_p, T_s, R_a, w_b, kpp, w_N, u_gN)


% Active power calculation
P = 3/2*real(u_c_ref*conj(i_c));

% Equation for grid angular frequency
w_g = (P_ref - P)*K_p + w_N;

% Update (integrate) the grid voltage angle
if(enabled==true)
    theta_next = theta + T_s * w_g;
else
     theta_next = theta_pll + T_s * w_g;
end

while(theta_next > pi)
    theta_next = theta_next - 2*pi;
end
while(theta_next < -pi)
    theta_next = theta_next + 2*pi;
end

% Extracting the real and imaginary values of the complex converter current
i_c_imag = imag(i_c);

% Applying lowpass filter equation to imaginary part of the
% converter current and forming reference current based on power reference
if(enabled==true)
    i_c_filt_next =  i_c_filt*(1 - w_b*T_s) + i_c_imag*(w_b*T_s);
else
    i_c_filt_next = i_c_filt;
end
i_ref = P_ref/(u_gN*kpp) + 1j*i_c_filt_next;

% Equation for reference voltage
u_c = u_gN + (i_ref-i_c) * R_a;

% Inverse coordinate transformation
u_cs = u_c*exp(1j*(theta + 1.5 * T_s * w_g));

== matlab function rfpsc_parallel/Grid inductance and load/MATLAB Function ==
  data: i_c1 input; i_c2 input; breaker2 input; breaker1 input; u_pcc output; u_c2 input; L_g parameter; L_f1 parameter; L_f2 parameter; u_c1 input; R_L input; R_f1 parameter; R_f2 parameter
function u_pcc = fcn(i_c1, i_c2, breaker2, breaker1, u_c2, L_g, L_f1, L_f2, u_c1, R_L, R_f1, R_f2)
u_pcc = 0;
if(breaker2 == 1 && breaker1 == 1)
    u_pcc = (L_g/L_f1*(u_c1-R_f1*i_c1) + L_g/L_f2*(u_c2-R_f2*i_c2) + R_L*(i_c1+i_c2))/(1 + L_g/L_f1 + L_g/L_f2);
elseif(breaker2 == 0 && breaker1 == 1)
    u_pcc = (L_g/L_f1*(u_c1+(R_f1+R_L)*i_c1))/(1 + L_g/L_f1);
elseif(breaker2 == 1 && breaker1 == 0)
     u_pcc = (L_g/L_f2*(u_c2+(R_f2+R_L)*i_c2))/(1 + L_g/L_f2);
end

== matlab function rfpsc_parallel/Grid inductance and load/MATLAB Function1 ==
  data: u_abc input size=3; u_s output size=1
function u_s = abc2s(u_abc)

% Space-vector transformation
u_s = 2/3*(u_abc(1) + u_abc(2)*exp(1j*2*pi/3) + u_abc(3)*exp(1j*4*pi/3));

== matlab function rfpsc_parallel/Grid inductance and load/MATLAB Function2 ==
  data: u_abc input size=3; u_s output size=1
function u_s = abc2s(u_abc)

% Space-vector transformation
u_s = 2/3*(u_abc(1) + u_abc(2)*exp(1j*2*pi/3) + u_abc(3)*exp(1j*4*pi/3));

== matlab function rfpsc_parallel/Grid inductance and load/MATLAB Function3 ==
  data: u_s input size=1; u_abc output size=3
function u_abc = s2abc(u_s)

% Inverse space-vector transformation
u_abc = real([1; exp(-1j*2*pi/3); exp(-1j*4*pi/3)]*u_s);

== matlab function rfpsc_parallel/Grid inductance and load/MATLAB Function4 ==
  data: i_s input size=1; i_abc output size=3
function i_abc = s2abc(i_s)

% Inverse space-vector transformation
i_abc = real([1; exp(-1j*2*pi/3); exp(-1j*4*pi/3)]*i_s);

== matlab function rfpsc_parallel/MATLAB Function3 ==
  data: y_alpha input double; y_dq output double; y_beta input double; theta input
function y_dq = fcn(y_alpha, y_beta, theta)

% Coordinate Transformation (Alpha-beta to dq)
y_s = y_alpha + 1j*y_beta;
y_dq = y_s * exp(-1j*theta);

== matlab function rfpsc_parallel/RFPSC2/PWM/MATLAB Function ==
  data: d_abc output double; u_cs_ref input; u_dc input; U_dcmin parameter
function d_abc = PWM(u_cs_ref, u_dc, U_dcmin)

%% Symmetrical suboscillation PWM
% Components of the voltage space vector
u_c_alpha_ref = real(u_cs_ref);
u_c_beta_ref  = imag(u_cs_ref);

% Phase-voltage references
u_ca_ref = u_c_alpha_ref;
u_cb_ref = .5*(-u_c_alpha_ref + sqrt(3)*u_c_beta_ref);
u_cc_ref = .5*(-u_c_alpha_ref - sqrt(3)*u_c_beta_ref);

% Vector of phase-voltage references
u_c_abc_ref = [u_ca_ref; u_cb_ref; u_cc_ref];

% Symmetrization of the references by adding the zero-sequence voltage
u0 = .5*(max(u_c_abc_ref) + min(u_c_abc_ref));
u_c_abc_ref = u_c_abc_ref - u0;

if (u_dc>=U_dcmin)
    % Clipping of the reference voltages such that no phase error is caused. 
    % If all phase voltage reference are realizable (below u_dc/2), m = 1 holds.
    m = max([2.*u_c_abc_ref./u_dc; 1]);
    u_c_abc_ref = u_c_abc_ref./m;
    
    % Duty cycles, which can be directly used for triangle comparison, 
    % if the triangle wave varies between 0...1
    d_abc = .5 + u_c_abc_ref./u_dc;
else
    d_abc = [0; 0; 0];
end

% % Realized voltage vector is calculated from the clamped duty ratios.
% % If the PWM does not saturate, u_c_ref_lim = u_c_ref holds. The realized
% % voltage vector is needed, e.g., for the current-controller antiwindup.
% u_cs_ref_lim = 2/3*(d_abc(1) + d_abc(2)*exp(1j*2*pi/3) ...
%     + d_abc(3)*exp(1j*4*pi/3))*u_dc;
% % In estimated rotor flux coordinates
% u_c_ref_lim = exp(-1j*theta)*u_cs_ref_lim;

== matlab function rfpsc_parallel/L_f1/MATLAB Function ==
  data: u_c_abc input; u_pcc_abc input; u_c_s output; u_pcc_s output
function [u_c_s, u_pcc_s] = abc2s(u_c_abc, u_pcc_abc)

% Space Vector Transformation of converter and pcc voltage
u_c_s = 2/3*(u_c_abc(1) + u_c_abc(2)*exp(1j*2*pi/3) + u_c_abc(3)*exp(1j*4*pi/3));

u_pcc_s = 2/3*(u_pcc_abc(1) + u_pcc_abc(2)*exp(1j*2*pi/3) + u_pcc_abc(3)*exp(1j*4*pi/3));

== matlab function rfpsc_parallel/RFPSC2/Reference Voltage Limiter/MATLAB Function ==
  data: d_abc input; u_dc input; u_c_ref_lim output; theta input; w_N parameter; T_s parameter
function u_c_ref_lim = ref_lim(d_abc, u_dc, theta, w_N, T_s)

u_c_ref_lim = 0;
% % Realized voltage vector is calculated from the clamped duty ratios.
% % If the PWM does not saturate, u_c_ref_lim = u_c_ref holds. The realized
% % voltage vector is needed, e.g., for the current-controller antiwindup.
u_cs_ref_lim = 2/3*(d_abc(1) + d_abc(2)*exp(1j*2*pi/3) ...
    + d_abc(3)*exp(1j*4*pi/3))*u_dc;

% % In estimated rotor flux coordinates
u_c_ref_lim = exp(-1j*(theta + 1.5 * w_N * T_s)).*u_cs_ref_lim;

== matlab function rfpsc_parallel/RFPSC2/abc to dq transformation ==
  data: i_c output; i_c_abc input; theta input
function i_c = abc2dq(i_c_abc, theta)

% Space Vector Transformation (abc to alpha-beta)
i_cs = 2/3 * (i_c_abc(1) + i_c_abc(2)*exp(1j*2*pi/3) ... 
    + i_c_abc(3)*exp(1j*4*pi/3));

% Coordinate Transformation (Alpha-beta to dq)
i_c = i_cs * exp(-1j*theta);

== matlab function rfpsc_parallel/abc to dq transformation ==
  data: y_c output; y_c_abc input; theta input
function y_c = abc2dq(y_c_abc, theta)

% Space Vector Transformation (abc to alpha-beta)
i_cs = 2/3 * (y_c_abc(1) + y_c_abc(2)*exp(1j*2*pi/3) ... 
    + y_c_abc(3)*exp(1j*4*pi/3));

% Coordinate Transformation (Alpha-beta to dq)
y_c = i_cs * exp(-1j*theta);

== matlab function rfpsc_parallel/abc to dq transformation1 ==
  data: y_c output; y_c_abc input; theta input
function y_c = abc2dq(y_c_abc, theta)

% Space Vector Transformation (abc to alpha-beta)
i_cs = 2/3 * (y_c_abc(1) + y_c_abc(2)*exp(1j*2*pi/3) ... 
    + y_c_abc(3)*exp(1j*4*pi/3));

% Coordinate Transformation (Alpha-beta to dq)
y_c = i_cs * exp(-1j*theta);

== matlab function rfpsc_parallel/abc to dq transformation2 ==
  data: y_c output; y_c_abc input; theta input
function y_c = abc2dq(y_c_abc, theta)

% Space Vector Transformation (abc to alpha-beta)
i_cs = 2/3 * (y_c_abc(1) + y_c_abc(2)*exp(1j*2*pi/3) ... 
    + y_c_abc(3)*exp(1j*4*pi/3));

% Coordinate Transformation (Alpha-beta to dq)
y_c = i_cs * exp(-1j*theta);

== matlab function rfpsc_parallel/abc to dq transformation3 ==
  data: y_c output; y_c_abc input; theta input
function y_c = abc2dq(y_c_abc, theta)

% Space Vector Transformation (abc to alpha-beta)
i_cs = 2/3 * (y_c_abc(1) + y_c_abc(2)*exp(1j*2*pi/3) ... 
    + y_c_abc(3)*exp(1j*4*pi/3));

% Coordinate Transformation (Alpha-beta to dq)
y_c = i_cs * exp(-1j*theta);

== matlab function rfpsc_parallel/MATLAB Function4 ==
  data: i_c input; u_c input; P output
function P = fcn(i_c, u_c)

P = 3/2*real((u_c)*conj(i_c));

== matlab function rfpsc_parallel/MATLAB Function5 ==
  data: u_hat output; i_g input; p_c1 input; p_hat output; p_c2 input; q_hat output
function [u_hat, p_hat, q_hat]  = fcn(i_g, p_c1, p_c2)

p_hat = p_c1 + p_c2;
u_hat_d = 2*p_hat/(3*real(i_g));
q_hat = -3/2*u_hat_d*imag(i_g);
u_hat = u_hat_d + 1j*0;

== matlab function rfpsc_parallel/MATLAB Function7 ==
  data: i_c input; u_c input; Q output
function Q = fcn(i_c, u_c)

Q = 3/2*imag((u_c)*conj(i_c));

== matlab function rfpsc_parallel/MATLAB Function8 ==
  data: i_c input; u_c input; Q output
function Q = fcn(i_c, u_c)

Q = 3/2*imag((u_c)*conj(i_c));

== matlab function rfpsc_parallel/Scaler /PWM/MATLAB Function ==
  data: d_abc output; u_cs_ref input; u_dc input
function d_abc = PWM(u_cs_ref, u_dc)

%% Symmetrical suboscillation PWM
% Components of the voltage space vector
u_c_alpha_ref = real(u_cs_ref);
u_c_beta_ref  = imag(u_cs_ref);

% Phase-voltage references
u_ca_ref = u_c_alpha_ref;
u_cb_ref = .5*(-u_c_alpha_ref + sqrt(3)*u_c_beta_ref);
u_cc_ref = .5*(-u_c_alpha_ref - sqrt(3)*u_c_beta_ref);

% Vector of phase-voltage references
u_c_abc_ref = [u_ca_ref; u_cb_ref; u_cc_ref];

% Symmetrization of the references by adding the zero-sequence voltage
u0 = .5*(max(u_c_abc_ref) + min(u_c_abc_ref));
u_c_abc_ref = u_c_abc_ref - u0;

% Clipping of the reference voltages such that no phase error is caused. 
% If all phase voltage reference are realizable (below u_dc/2), m = 1 holds.
m = max([2*u_c_abc_ref/u_dc; 1]);
u_c_abc_ref = u_c_abc_ref/m;

% Duty cycles, which can be directly used for triangle comparison, 
% if the triangle wave varies between 0...1
d_abc = .5 + u_c_abc_ref/u_dc;

== matlab function rfpsc_parallel/Scaler /RFPSC/RFPSC ==
  data: i_c input; P_ref input; u_cs output double; theta_next output; w_1 input; V input; u_c_ref input; K_p input; R_a input; theta input; i_c_filt input; T_s parameter; i_c_filt_next output double; w_b parameter; kpp parameter
function [u_cs, theta_next, i_c_filt_next] = ... 
    RFPSC(i_c, P_ref, w_1, V, u_c_ref, K_p, R_a, theta, i_c_filt, ... 
    T_s, w_b, kpp)


% Active power calculation
P = kpp*real(u_c_ref*conj(i_c));

% Equation for grid angular frequency
w_g = (P_ref - P)*K_p + w_1;

% Update (integrate) the grid voltage angle
theta_next = theta + T_s * w_g;
if(theta_next > pi)
    theta_next = theta_next - 2*pi;
elseif(theta_next < -pi)
    theta_next = theta_next + 2*pi;
end

% Extracting the real and imaginary values of the complex converter current
i_c_imag = imag(i_c);

% Applying lowpass filter equation to imaginary part of the
% converter current and forming reference current based on power reference
i_c_filt_next =  i_c_filt*(1 - w_b*T_s) + i_c_imag*(w_b*T_s);

%if(V == 0 || kpp == 0)
%    i_ref = i_c;
%else    
    i_ref = P_ref/(V*kpp) + 1j*i_c_filt_next;
%end

% Equation for reference voltage
u_c = V + (i_ref-i_c) * R_a;

% Inverse coordinate transformation
u_cs = u_c*exp(1j*(theta + 1.5 * T_s * w_g));

== matlab function rfpsc_parallel/Scaler /Reference Voltage Limiter/MATLAB Function ==
  data: d_abc input; u_dc input; u_c_ref_lim output; theta input; w_g parameter; T_s parameter
function u_c_ref_lim = ref_lim(d_abc, u_dc, theta, w_g, T_s)

% % Realized voltage vector is calculated from the clamped duty ratios.
% % If the PWM does not saturate, u_c_ref_lim = u_c_ref holds. The realized
% % voltage vector is needed, e.g., for the current-controller antiwindup.
u_cs_ref_lim = 2/3*(d_abc(1) + d_abc(2)*exp(1j*2*pi/3) ...
    + d_abc(3)*exp(1j*4*pi/3))*u_dc;

% % In estimated rotor flux coordinates
u_c_ref_lim = exp(-1j*(theta + 1.5 * w_g * T_s))*u_cs_ref_lim;

== matlab function rfpsc_parallel/Scaler /abc to dq transformation ==
  data: i_c output; i_c_abc input; theta input
function i_c = abc2dq(i_c_abc, theta)

% Space Vector Transformation (abc to alpha-beta)
i_cs = 2/3 * (i_c_abc(1) + i_c_abc(2)*exp(1j*2*pi/3) ... 
    + i_c_abc(3)*exp(1j*4*pi/3));

% Coordinate Transformation (Alpha-beta to dq)
i_c = i_cs * exp(-1j*theta);

== matlab function rfpsc_parallel/L_f2/MATLAB Function ==
  data: u_c_abc input; u_pcc_abc input; u_c_s output; u_pcc_s output
function [u_c_s, u_pcc_s] = abc2s(u_c_abc, u_pcc_abc)

% Space Vector Transformation of converter and pcc voltage
u_c_s = 2/3*(u_c_abc(1) + u_c_abc(2)*exp(1j*2*pi/3) + u_c_abc(3)*exp(1j*4*pi/3));

u_pcc_s = 2/3*(u_pcc_abc(1) + u_pcc_abc(2)*exp(1j*2*pi/3) + u_pcc_abc(3)*exp(1j*4*pi/3));

== matlab function rfpsc_parallel/RFPSC2/PLL/PLL ==
  data: u_g_abc input size=3; theta_g input double; w_gi input double; u_gN parameter; w0_pll parameter; theta_g_new output double; w_gi_new output double; T_s parameter
function [theta_g_new, w_gi_new] = pll(u_g_abc, ...
    theta_g, w_gi, u_gN, w0_pll, T_s)

%theta_g_new = 0;

% Parameters 
% (Tuning of the PLL is analogous to that of the DC-voltage controller.)
zeta = 1;   % Damping ratio
k_p = 2*zeta*w0_pll/u_gN; 
k_i = w0_pll^2/u_gN;

% Space-vector transformation from phase voltages
u_gs = 2/3*(u_g_abc(1) + u_g_abc(2)*exp(1j*2*pi/3) + u_g_abc(3)*exp(1j*4*pi/3));

% Coordinate transformation to the "estimated" grid coordinates
u_g = u_gs*exp(-1j*theta_g);

% Error signal, which is drive to zero by the PLL
u_gq = imag(u_g);

w_g = k_p*u_gq + w_gi;

% Update the integral state
w_gi_new = w_gi + T_s*k_i*u_gq;

% Update the grid-voltage angle
theta_g_new = theta_g + T_s*w_g;
while(theta_g_new > pi)
    theta_g_new = theta_g_new - 2*pi;
end
while(theta_g_new < -pi)
    theta_g_new = theta_g_new + 2*pi;
end
